simulink model "Practica1.1"  (R2025b)
settings: Solver=VariableStepAuto  StartTime=0.0  StopTime=10  MaxStep=1e-3  RelTol=1e-3
settings Model: Creator=jlope

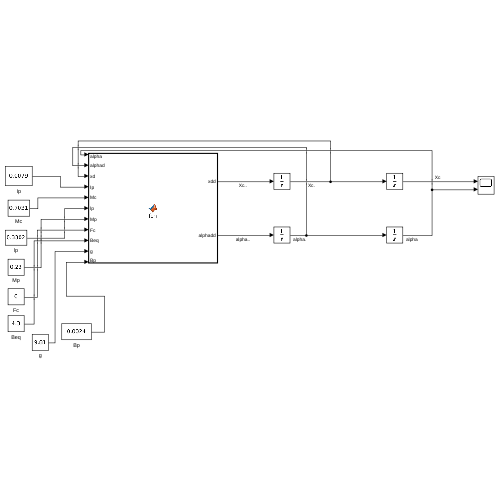
[thumbnail: Simulink's stored preview of the top-level diagram]
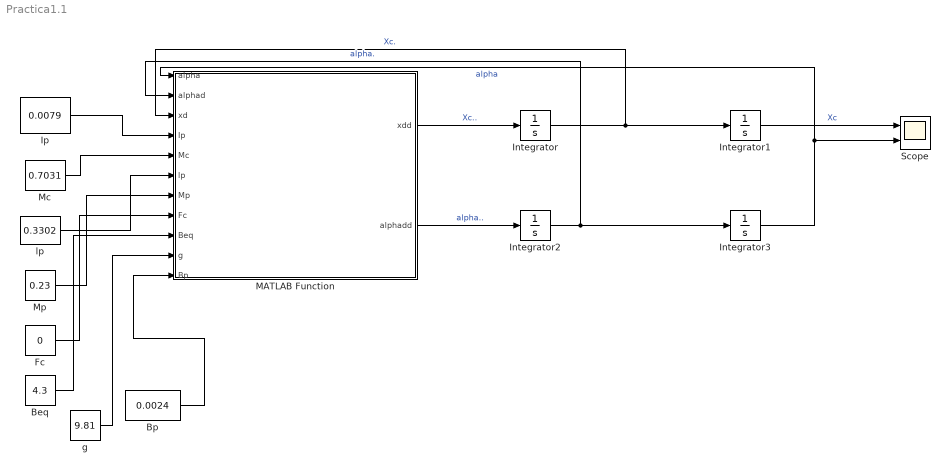
== system Practica1.1 ==
  Beq : Constant  Value=4.3
  Bp : Constant  Value=0.0024
  Fc : Constant  Value=0
  Integrator : Integrator
  Integrator1 : Integrator
  Integrator2 : Integrator
  Integrator3 : Integrator  InitialCondition=1*(pi/180)
  Ip : Constant  Value=0.0079
  MATLAB Function : MATLAB Function  TreatAsAtomicUnit=on
  Mc : Constant  Value=0.7031
  Mp : Constant  Value=0.23
  Scope : Scope  NumInputPorts=2
      settings: ActiveDisplayYMinimum=-0.019318550311866314  ActiveDisplayYMaximum=0.17386695280679687
  g : Constant  Value=9.81
  lp : Constant  Value=0.3302
  wires:
  Integrator/1 -> MATLAB Function/3(xd), Integrator1/1  "Xc."
  Integrator1/1 -> Scope/1  "Xc"
  MATLAB Function/1(xdd) -> Integrator/1  "Xc.."
  MATLAB Function/2(alphadd) -> Integrator2/1  "alpha.."
  Integrator2/1 -> Integrator3/1, MATLAB Function/2(alphad)  "alpha."
  Integrator3/1 -> MATLAB Function/1(alpha), Scope/2  "alpha"
  Fc/1 -> MATLAB Function/8(Fc)
  Ip/1 -> MATLAB Function/4(Ip)
  Mc/1 -> MATLAB Function/5(Mc)
  lp/1 -> MATLAB Function/6(lp)
  Mp/1 -> MATLAB Function/7(Mp)
  Beq/1 -> MATLAB Function/9(Beq)
  g/1 -> MATLAB Function/10(g)
  Bp/1 -> MATLAB Function/11(Bp)

== matlab function Practica1.1/MATLAB Function ==
  data: alpha input; alphad input; xd input; Ip input; Mc input; lp input; Mp input; Fc input; xdd output; alphadd output; Beq input; g input; Bp input
function [xdd, alphadd] = fcn(alpha, alphad, xd,Ip,Mc,lp,Mp,Fc,Beq,g,Bp)

den = (Mc + Mp)*Ip + Mc*Mp*(lp^2) + (Mp^2)*(lp^2)*(sin(alpha)^2);

Num_x = (Ip + Mp*lp^2)*Fc ...
      + Mp^2 * lp^2 * g * cos(alpha) * sin(alpha) ...
      - (Ip + Mp*lp^2) * Beq * xd ...
      - (Ip*Mp*lp - Mp^2*lp^3) * (alphad^2) * sin(alpha) ...
      - Mp * lp * alphad * cos(alpha) * Bp;

xdd = Num_x / den;

Num_a = (Mc + Mp) * Mp * g * lp * sin(alpha) ...
      - (Mc + Mp) * Bp * alphad ...
      + Fc * Mp * lp * cos(alpha) ...
      - Mp^2 * lp^2 * (alphad^2) * sin(alpha) * cos(alpha) ...
      - Beq * Mp * lp * xd * cos(alpha);

alphadd = Num_a / den;
